simulink model "validating_pid_controller"  (R2012b)
settings: Solver=ode45  StartTime=0.0  StopTime=1  RelTol=1e-3
undefined symbols (not defined in the file): C, Cd, G, Gd, Ts
settings Model: Creator=Juliano  LastModifiedBy=Juliano

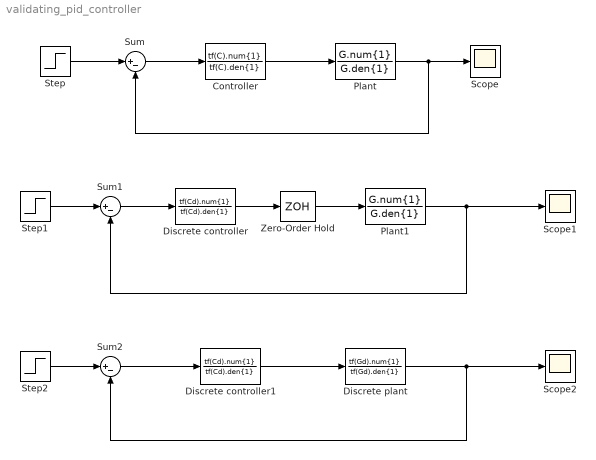
== system validating_pid_controller ==
  Controller : TransferFcn  Numerator=tf(C).num{1}  Denominator=tf(C).den{1}
  Discrete controller : DiscreteTransferFcn  Numerator=tf(Cd).num{1}  Denominator=tf(Cd).den{1}  SampleTime=Ts
  Discrete controller1 : DiscreteTransferFcn  Numerator=tf(Cd).num{1}  Denominator=tf(Cd).den{1}  SampleTime=Ts
  Discrete plant : DiscreteTransferFcn  Numerator=tf(Gd).num{1}  Denominator=tf(Gd).den{1}  SampleTime=Ts
  Plant : TransferFcn  Numerator=G.num{1}  Denominator=G.den{1}
  Plant1 : TransferFcn  Numerator=G.num{1}  Denominator=G.den{1}
  Scope : Scope
  Scope1 : Scope
  Scope2 : Scope
      settings: SaveName=ScopeData2
  Step : Step  Time=0  SampleTime=0
  Step1 : Step  Time=0  SampleTime=0
  Step2 : Step  Time=0  SampleTime=0
  Sum : Sum  Inputs=|+-
  Sum1 : Sum  Inputs=|+-
  Sum2 : Sum  Inputs=|+-
  Zero-Order Hold : ZeroOrderHold  SampleTime=Ts
  wires:
  Step/1 -> Sum/1
  Step1/1 -> Sum1/1
  Sum1/1 -> Discrete controller/1
  Sum/1 -> Controller/1
  Controller/1 -> Plant/1
  Plant/1 -> Sum/2, Scope/1
  Discrete controller/1 -> Zero-Order Hold/1
  Zero-Order Hold/1 -> Plant1/1
  Plant1/1 -> Sum1/2, Scope1/1
  Step2/1 -> Sum2/1
  Sum2/1 -> Discrete controller1/1
  Discrete plant/1 -> Scope2/1, Sum2/2
  Discrete controller1/1 -> Discrete plant/1
